simulink model "HeadCtrl_PI"  (R2017a)
settings: Solver=FixedStepDiscrete  StartTime=0.0  StopTime=10  FixedStep=0.01  RelTol=1e-3
PreLoadFcn:
  | robotParameters;
undefined symbols (not defined in the file or in its folder): axleLength, motorIp, motorSp, ticksPerRot, wheelR
libraries: mobileRoboticsTrainingLib x5, simulink x1, simulink_extras x1
settings Model: Creator=sseshadr  LastModifiedBy=shiremat

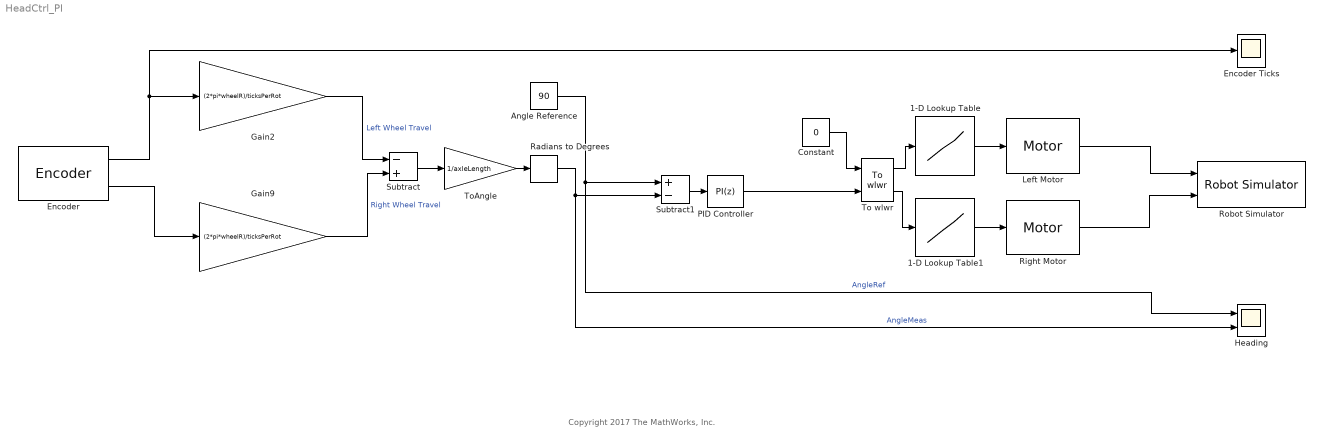
== system HeadCtrl_PI ==
  note: Copyright 2017 The MathWorks, Inc.
  1-D Lookup Table : Lookup_n-D  NumberOfTableDimensions=1  BreakpointsForDimension1=motorSp  Table=motorIp  ExtrapMethod=Clip  InternalRulePriority=Speed  RndMeth=Simplest  InputSameDT=on
  1-D Lookup Table1 : Lookup_n-D  NumberOfTableDimensions=1  BreakpointsForDimension1=motorSp  Table=motorIp  ExtrapMethod=Clip  InternalRulePriority=Speed  RndMeth=Simplest  InputSameDT=on
  Angle Reference : Constant  Value=90
  Constant : Constant  Value=0
  Encoder : mobileRoboticsTrainingLib/Encoder  axleLength=axleLength  wheelR=wheelR  ticksPerRot=1
      settings: SourceProductName=Mobile Robotics Training Library
  Encoder Ticks : Scope
  Gain2 : Gain  Gain=(2*pi*wheelR)/ticksPerRot
  Gain9 : Gain  Gain=(2*pi*wheelR)/ticksPerRot
  Heading : Scope  NumInputPorts=2
  Left Motor : mobileRoboticsTrainingLib/Motor  motorPlant=wheelMotorModel  sensorType=Speed
      settings: SourceProductName=Mobile Robotics Training Library
  PID Controller : simulink/Continuous/PID Controller  Controller=PI  TimeDomain=Discrete-time  SampleTime=-1  IntegratorMethod=Forward Euler  FilterMethod=Forward Euler  Form=Parallel  UseFilter=off  ControllerParametersSource=internal  P=0.1  I=0.001  D=-0.0140783779685636  N=151.701833251505  InitialConditionSource=internal  InitialConditionForIntegrator=0  InitialConditionForFilter=0  ExternalReset=none  LimitOutput=on  UpperSaturationLimit=4  LowerSaturationLimit=-4  LinearizeAsGain=on  AntiWindupMode=clamping  Kb=1  TrackingMode=off  Kt=1  PParamMin=[]  PParamMax=[]  IParamMin=[]  IParamMax=[]  DParamMin=[]  DParamMax=[]  NParamMin=[]  NParamMax=[]  KbParamMin=[]  KbParamMax=[]  KtParamMin=[]  KtParamMax=[]  POutMin=[]  POutMax=[]  IOutMin=[]  IOutMax=[]  DOutMin=[]  DOutMax=[]  NOutMin=[]  NOutMax=[]  KbOutMin=[]  KbOutMax=[]  KtOutMin=[]  KtOutMax=[]  IntegratorOutMin=[]  IntegratorOutMax=[]  FilterOutMin=[]  FilterOutMax=[]  SumOutMin=[]  SumOutMax=[]  SumI1OutMin=[]  SumI1OutMax=[]  SumI2OutMin=[]  SumI2OutMax=[]  SumI3OutMin=[]  SumI3OutMax=[]  SumDOutMin=[]  SumDOutMax=[]  SaturationOutMin=[]  SaturationOutMax=[]  IntegratorContinuousStateAttributes=''  IntegratorStateMustResolveToSignalObject=off  IntegratorRTWStateStorageClass=Auto  FilterContinuousStateAttributes=''  FilterStateMustResolveToSignalObject=off  FilterRTWStateStorageClass=Auto  DifferentiatorICPrevScaledInput=0  DifferentiatorOutMin=[]  DifferentiatorOutMax=[]  InitialConditionSetting=Output
  Radians to Degrees : simulink_extras/Transformations/Radians to Degrees
  Right Motor : mobileRoboticsTrainingLib/Motor  motorPlant=wheelMotorModel  sensorType=Speed
      settings: SourceProductName=Mobile Robotics Training Library
  Robot Simulator : mobileRoboticsTrainingLib/Robot Simulator  Priority=99  mapVar=[]  startX=2  startY=2  startTheta=0  axleLength=axleLength  wheelR=wheelR
  Subtract : Sum  Inputs=-+
  Subtract1 : Sum  Inputs=+-
  To wlwr : mobileRoboticsTrainingLib/To wlwr  axleLength=0.1  wheelR=0.05
  ToAngle : Gain  Gain=1/axleLength
  wires:
  Radians to Degrees/1 -> Subtract1/2, Heading/2  "AngleMeas"
  Gain2/1 -> Subtract/1  "Left Wheel Travel"
  Subtract/1 -> ToAngle/1
  Gain9/1 -> Subtract/2  "Right Wheel Travel"
  Encoder/1 -> Gain2/1, Encoder Ticks/1
  Encoder/2 -> Gain9/1
  To wlwr/1 -> 1-D Lookup Table/1
  1-D Lookup Table/1 -> Left Motor/1
  1-D Lookup Table1/1 -> Right Motor/1
  Left Motor/1 -> Robot Simulator/1
  To wlwr/2 -> 1-D Lookup Table1/1
  Right Motor/1 -> Robot Simulator/2
  Angle Reference/1 -> Subtract1/1, Heading/1  "AngleRef"
  ToAngle/1 -> Radians to Degrees/1
  PID Controller/1 -> To wlwr/2
  Constant/1 -> To wlwr/1
  Subtract1/1 -> PID Controller/1
